simulink model "GPCA_System_Monitor"  (Simulink 8.7)
settings: Solver=VariableStepAuto  StartTime=0.0  StopTime=10.0  RelTol=1e-3
libraries: simulink x1
settings Model: Creator=bourbouh  LastModifiedBy=bourbouh
settings DataIOCC: LimitDataPoints=off  SaveFormat=Dataset
settings DebuggingCC: UnderspecifiedInitializationDetection=Simplified  MergeDetectMultiDrivingBlocksExec=error
settings HardwareCC: ProdBitPerPointer=64  ProdLargestAtomicFloat=Float  ProdIntDivRoundTo=Zero  ProdEndianess=LittleEndian  ProdWordSize=64  ProdHWDeviceType=Intel->x86-64 (Windows64)
settings ModelReferenceCC: PropagateSignalLabelsOutOfModel=on
settings ConfigComp: CovModelRefEnable=off

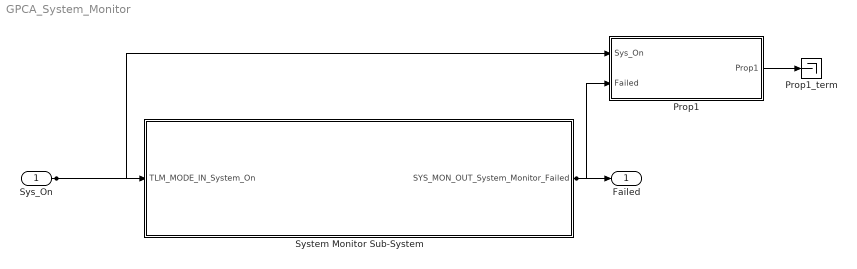
== system GPCA_System_Monitor ==
  Sys_On : Inport
  Prop1 : Subsystem  TreatAsAtomicUnit=on  mask(Observer){AnnotationType=ensures, ObserverType=[]}
      mask prompts: AnnotationType "Type of annotation (pre/post...)"; ObserverType "Observer type"
      mask help:
      | Set an observer for the system.
      | The annotation type parameter sets the type of observer:
      | - requires : pre-condition
      | - ensures : post-condition
      | - assert : an assertion
      | - observer : the observer computes a special type of properties
      mask TypeOptions AnnotationType: ensures | requires | assert | observer
      mask Callback AnnotationType:
      | paramStr = get_param(gcb, 'MaskValues');
      | if strcmp(paramStr{1}(1),'o')
      | set_param(gcb,'MaskVisibilities',{'on';'on'});
      | paramStr{2} = 'ellipsoid';
      | set_param(gcb,'MaskValues',paramStr);
      | else
      | set_param(gcb,'MaskVisibilities',{'on';'off'});
      | end
      | clear paramStr;
      mask Callback ObserverType:
      | paramStr = get_param(gcb, 'MaskValues');
      | if strcmp(paramStr{1}(1),'o')
      | set_param(gcb,'MaskVisibilities',{'on';'on'});
      | paramStr{2} = 'ellipsoid';
      | set_param(gcb,'MaskValues',paramStr);
      | else
      | set_param(gcb,'MaskVisibilities',{'on';'off'});
      | end
      | clear paramStr;
      mask Display:
      | color('black')
      | text(0.5, 0.5, ['Property: ''' get_param(gcb,'name') ''''], 'horizontalAlignment', 'center');
      | text(0.99, 0.03, '{\bf\fontsize{12}SAFE}', 'hor', 'right', 'ver', 'bottom', 'texmode', 'on');
  Prop1_term : Terminator
  System Monitor Sub-System : Stateflow chart  TreatAsAtomicUnit=on
  Failed : Outport
  wires:
  Sys_On/1 -> System Monitor Sub-System/1(TLM_MODE_IN_System_On), Prop1/1(Sys_On)
  System Monitor Sub-System/1(SYS_MON_OUT_System_Monitor_Failed) -> Failed/1, Prop1/2(Failed)
  Prop1/1(Prop1) -> Prop1_term/1

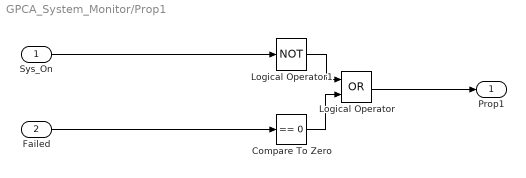
== system GPCA_System_Monitor/Prop1 ==
  Sys_On : Inport
  Failed : Inport  Port=2
  Compare To Zero : simulink/Logic and Bit Operations/Compare To Zero  relop===  OutDataTypeStr=boolean
  Logical Operator : Logic  Operator=OR  AllPortsSameDT=off  OutDataTypeStr=boolean
  Logical Operator1 : Logic  Operator=NOT  AllPortsSameDT=off  OutDataTypeStr=boolean
  Prop1 : Outport
  wires:
  Sys_On/1 -> Logical Operator1/1
  Failed/1 -> Compare To Zero/1
  Logical Operator/1 -> Prop1/1
  Logical Operator1/1 -> Logical Operator/1
  Compare To Zero/1 -> Logical Operator/2

== stateflow chart System Monitor Sub-System ==
  state System_Monitor
    entry: SYS_MON_OUT_System_Monitor_Failed=0;
    during: SYS_MON_OUT_System_Monitor_Failed=0;
    exit: SYS_MON_OUT_System_Monitor_Failed=0;
  state NOT_ON
  (default) -> System_Monitor [order 1] : [TLM_MODE_IN_System_On]
  (default) -> NOT_ON [order 2]
  NOT_ON -> System_Monitor : [TLM_MODE_IN_System_On]
  System_Monitor -> NOT_ON : [!TLM_MODE_IN_System_On]
  data: TLM_MODE_IN_System_On input boolean; SYS_MON_OUT_System_Monitor_Failed output boolean
